simulink model "DroneNonLinearController"  (R2021a)
settings: Solver=VariableStepAuto  StartTime=0.0  StopTime=100  RelTol=1e-3
settings Model: Creator=aruna  LastModifiedBy=aruna

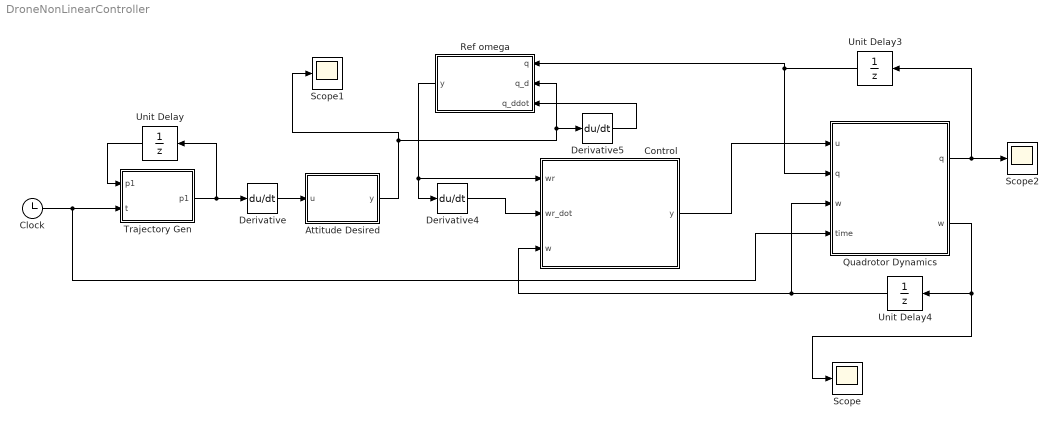
== system DroneNonLinearController ==
  Attitude Desired : MATLAB Function  TreatAsAtomicUnit=on
  Clock : Clock
  Control : MATLAB Function  TreatAsAtomicUnit=on
  Derivative : Derivative
  Derivative4 : Derivative
  Derivative5 : Derivative
  Quadrotor Dynamics : MATLAB Function  TreatAsAtomicUnit=on
  Ref omega : MATLAB Function  TreatAsAtomicUnit=on
  Scope : Scope
  Scope1 : Scope
  Scope2 : Scope
  Trajectory Gen : MATLAB Function  TreatAsAtomicUnit=on
  Unit Delay : UnitDelay  SampleTime=-1  HasFrameUpgradeWarning=on
  Unit Delay3 : UnitDelay  SampleTime=-1  HasFrameUpgradeWarning=on
  Unit Delay4 : UnitDelay  SampleTime=-1  HasFrameUpgradeWarning=on
  wires:
  Clock/1 -> Quadrotor Dynamics/4(time), Trajectory Gen/2(t)
  Trajectory Gen/1(p1) -> Derivative/1, Unit Delay/1
  Unit Delay/1 -> Trajectory Gen/1("p1 ")
  Derivative/1 -> Attitude Desired/1(u)
  Attitude Desired/1(y) -> Scope1/1, Derivative5/1, Ref omega/2(q_d)
  Quadrotor Dynamics/1(q) -> Scope2/1, Unit Delay3/1
  Quadrotor Dynamics/2(w) -> Scope/1, Unit Delay4/1
  Ref omega/1(y) -> Control/1(wr), Derivative4/1
  Derivative4/1 -> Control/2(wr_dot)
  Derivative5/1 -> Ref omega/3(q_ddot)
  Control/1(y) -> Quadrotor Dynamics/1(u)
  Unit Delay3/1 -> Ref omega/1(q), Quadrotor Dynamics/2("q ")
  Unit Delay4/1 -> Quadrotor Dynamics/3("w "), Control/3(w)

== matlab function DroneNonLinearController/Trajectory Gen ==
  data: p1 input size=[6,1]; t input; p1 output
function p1 = fcn(p1, t)
dt = 0.1;
time = t;

present_state = p1;
%p1 vector contains the position and velocity
x_present = [present_state(1);present_state(2)];
y_present = [present_state(3);present_state(4)];
z_present = [present_state(5);present_state(6)];

x_presentplus1 = rk4singlestep(@(time,x)x_pos(time,x),dt,time,x_present);
x_present = x_presentplus1;

y_presentplus1 = rk4singlestep(@(time,y)y_pos(time,y),dt,time,y_present);
y_present = y_presentplus1;

z_presentplus1 = rk4singlestep(@(time,z)z_pos(time,z),dt,time,z_present);
z_present = z_presentplus1;


p1 = vertcat(x_present,y_present,z_present);
end

function yout = rk4singlestep(fun,dt,tk,yk) 
f1 = fun(tk,yk);
f2 = fun(tk+dt/2,yk+(dt/2)*f1);
f3 = fun(tk+dt/2,yk+(dt/2)*f2);
f4 = fun(tk+dt,yk+dt*f3);

yout = yk + (dt/6)*(f1+2*f2+2*f3+f4);
end

function dx = x_pos(time,x)

dx = [x(2);4 - 3*x(2) - 2*x(1)];
end

function dy = y_pos(time,y)

dy = [y(2); 2 - 3*y(2) - 2*y(1)];
end

function dz = z_pos(time,z)

dz = [z(2);2 - 3*z(2) - 2*z(1)];
end

== matlab function DroneNonLinearController/Attitude Desired ==
  data: u input; y output
function y = fcn(u)


X_bar = u(2);
Y_bar = u(4);
Z_bar = u(6) + 9.81;

Fd = sqrt((X_bar)^2 + (Y_bar)^2 + (Z_bar)^2 );

psi_d = 0;
phi_d = asin(-(Y_bar)/Fd);
theta_d = atan2((X_bar)/Z_bar,1);

q_d = [theta_d;phi_d;psi_d];

y = q_d ;

== matlab function DroneNonLinearController/Control ==
  data: wr input size=[3,1]; y output; wr_dot input size=[3,1]; w input size=[3,1]
function y = fcn(wr, wr_dot, w)
J = [1 0 0; 0 1 0; 0 0 1];
K = 4.4.*[1 0 0; 0 1 0; 0 0 1];



cross = J*w;
cross_skew = [0 -cross(3) cross(2);cross(3) 0 -cross(1);-cross(2) cross(1) 0];
u = J*wr_dot - cross_skew*wr - K*(w - wr);

y = u;

== matlab function DroneNonLinearController/Quadrotor Dynamics ==
  data: u input; q input size=[3,1]; w input size=[3,1]; q output; w output; time input
function [q,w] = fcn(u, q, w, time)
dt = 0.36;
if time < 0.01
    w = [0;0;0];
    q = [0;0;0];
end

w_new = rk4singlestepat(@(w,u)omega(w,u),dt,w,u);
q_new = rk4singlestepat(@(q,w)attitude(q,w),dt,q,w);

w = w_new;
q = q_new;

end

function dw = omega(w,u)
J = [1 0 0;0 1 0;0 0 1];
omega = [w(1);w(2);w(3)];
cross = J*omega;
cross_skew = [0 -cross(3) cross(2);cross(3) 0 -cross(1);-cross(2) cross(1) 0];

dw = cross_skew*omega + u;
end

function dq = attitude(q,w)

theta = q(1);
phi = q(2);
psi = q(3);

Z_q = [1 sin(phi)*tan(theta) cos(phi)*tan(theta);0 cos(phi) -sin(phi);0 sin(phi)*sec(theta) cos(phi)*sec(theta)];
omega = [w(1);w(2);w(3)];
dq = Z_q*omega;
end

function yout = rk4singlestepat(fun,dt,yk,u) 
yk = [yk(1);yk(2);yk(3)];
f1 = fun(yk,u);
f2 = fun(yk+(dt/2)*f1,u);
f3 = fun(yk+(dt/2)*f2,u);
f4 = fun(yk+dt*f3,u);

yout = yk + (dt/6)*(f1+2*f2+2*f3+f4);
end

== matlab function DroneNonLinearController/Ref omega ==
  data: q input size=[3,1]; y output; q_d input; q_ddot input
function y = fcn(q, q_d, q_ddot)
theta = q(1);
phi = q(2);
psi = q(3);
att = [theta;phi;psi];
L = [1 0 0;0 1 0;0 0 1];%lambda parameter
J = [1 0 0;0 1 0;0 0 1];%inertia tensor

Z_q = [1 sin(phi)*tan(theta) cos(phi)*tan(theta);0 cos(phi) -sin(phi);0 sin(phi)*sec(theta) cos(phi)*sec(theta)];
w_r = Z_q\q_ddot + Z_q\L*(q_d - att);

y = w_r;
